simulink model "main"  (R2018a)
settings: Solver=VariableStepAuto  StartTime=0.0  StopTime=10  RelTol=1e-3
libraries: simulink x2
settings Model: Creator=user  LastModifiedBy=user

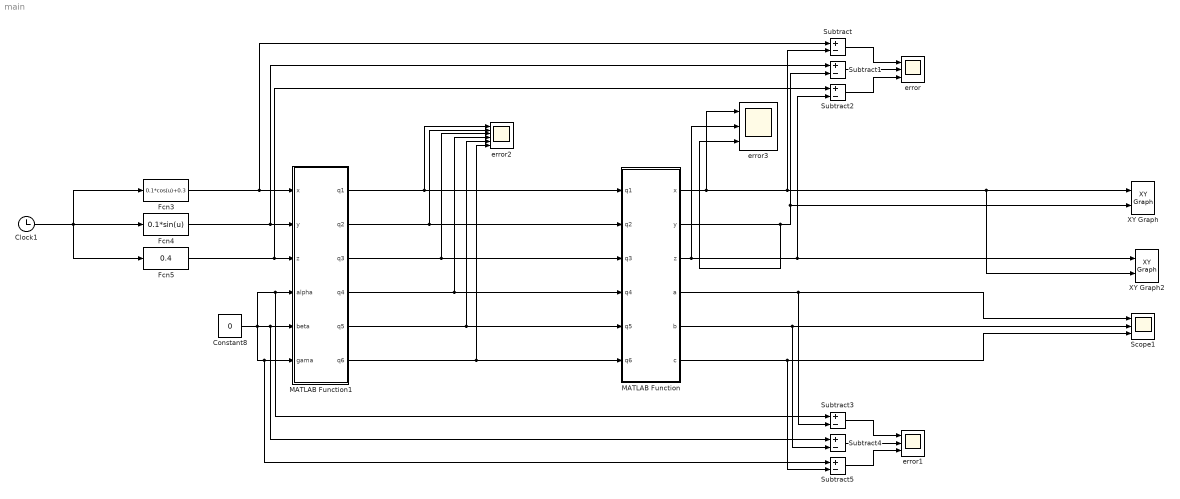
== system main ==
  Clock1 : Clock
  Constant8 : Constant  Value=0
  Fcn3 : Fcn  Expr=0.1*cos(u)+0.3
  Fcn4 : Fcn  Expr=0.1*sin(u)
  Fcn5 : Fcn  Expr=0.4
  MATLAB Function : MATLAB Function  TreatAsAtomicUnit=on
  MATLAB Function1 : MATLAB Function  TreatAsAtomicUnit=on
  Scope1 : Scope  NumInputPorts=3
  Subtract{,1..5} (6 alike) : Sum  Inputs=+-
  XY Graph : simulink/Sinks/XY Graph  xmin=-2  xmax=2  ymin=-2  ymax=2  st=-1
  XY Graph2 : simulink/Sinks/XY Graph  xmin=-2  xmax=2  ymin=-2  ymax=2  st=-1
  error : Scope  NumInputPorts=3
  error1 : Scope  NumInputPorts=3
  error2 : Scope  NumInputPorts=6
  error3 : Scope  NumInputPorts=3
  wires:
  Constant8/1 -> MATLAB Function1/4(alpha), Subtract3/1, MATLAB Function1/6(gama), Subtract5/1, MATLAB Function1/5(beta), Subtract4/1
  MATLAB Function/1(x) -> error3/1, Subtract/2, XY Graph2/2, XY Graph/1
  MATLAB Function/2(y) -> error3/3, Subtract1/2, XY Graph/2
  MATLAB Function/3(z) -> error3/2, XY Graph2/1, Subtract2/2
  MATLAB Function/4(a) -> Subtract3/2, Scope1/1
  MATLAB Function/5(b) -> Subtract4/2, Scope1/2
  MATLAB Function/6(c) -> Subtract5/2, Scope1/3
  MATLAB Function1/1(q1) -> error2/1, MATLAB Function/1(q1)
  Subtract/1 -> error/1
  Subtract1/1 -> error/2
  Subtract2/1 -> error/3
  Subtract5/1 -> error1/3
  Subtract4/1 -> error1/2
  Subtract3/1 -> error1/1
  MATLAB Function1/2(q2) -> error2/2, MATLAB Function/2(q2)
  MATLAB Function1/3(q3) -> error2/3, MATLAB Function/3(q3)
  MATLAB Function1/4(q4) -> error2/4, MATLAB Function/4(q4)
  MATLAB Function1/5(q5) -> error2/5, MATLAB Function/5(q5)
  Clock1/1 -> Fcn3/1, Fcn4/1, Fcn5/1
  MATLAB Function1/6(q6) -> error2/6, MATLAB Function/6(q6)
  Fcn3/1 -> Subtract/1, MATLAB Function1/1(x)
  Fcn4/1 -> Subtract1/1, MATLAB Function1/2(y)
  Fcn5/1 -> Subtract2/1, MATLAB Function1/3(z)

== matlab function main/MATLAB Function ==
  data: q1 input; x output; y output; z output; a output; b output; c output; q2 input; q3 input; q4 input; q5 input; q6 input
function [x,y,z,a,b,c] = FK(q1,q2,q3,q4,q5,q6)

% -------------DH_Parametrs--------------------
a0 = 0;     d1 = 0.352;      alpha0 = 0;
a1 = 0.07;    d2 = 0;        alpha1 = -pi/2;
a2 = 0.36;   d3 = 0;        alpha2 = 0;
a3 = 0;     d4 = 0.380;      alpha3 = -pi/2;
a4 = 0;     d5 = 0;        alpha4 = pi/2;
a5 = 0;     d6 = 0;        alpha5 = -pi/2;

theta1 =q1;
theta2 =q2;
theta3 =q3;
theta4 =q4; 
theta5 =q5;
theta6 =q6;


T10 = DHFUNCTION(a0,alpha0,d1,theta1);
T21 = DHFUNCTION(a1,alpha1,d2,(theta2-pi/2));
T32 = DHFUNCTION(a2,alpha2,d3,theta3);
T43 = DHFUNCTION(a3,alpha3,d4,theta4);
T54 = DHFUNCTION(a4,alpha4,d5,theta5);
T65 = DHFUNCTION(a5,alpha5,d6,theta6);

T20 = T10*T21;
T30 = T20*T32;
T64 = T54*T65;
T63 = T43*T64;
T60 = T30*T63;


Xw = T60(1,4);
Yw = T60(2,4);
Zw = T60(3,4);

P6 = [Xw;Yw;Zw];

PTCP= T60*[0;0;0.065;1];

x=PTCP(1);
y=PTCP(2);
z=PTCP(3);

a=atan2(sqrt(1-(T60(1,3)/sqrt(T60(1,3)^2+T60(2,3)^2+T60(3,3)^2))^2),T60(1,3)/sqrt(T60(1,3)^2+T60(2,3)^2+T60(3,3)^2));
b=atan2(sqrt(1-(T60(1,3)/sqrt(T60(1,3)^2+T60(2,3)^2+T60(3,3)^2))^2),T60(2,3)/sqrt(T60(1,3)^2+T60(2,3)^2+T60(3,3)^2));
c=atan2(sqrt(1-(T60(1,3)/sqrt(T60(1,3)^2+T60(2,3)^2+T60(3,3)^2))^2),T60(3,3)/sqrt(T60(1,3)^2+T60(2,3)^2+T60(3,3)^2));

function T = DHFUNCTION(ai,alphai,di,thetai)

T = [ cos(thetai), -1.*sin(thetai), 0, ai ;
 sin(thetai).*cos(alphai), cos(thetai).*cos(alphai), -1.*sin(alphai), 1*di.*sin(alphai);
 sin(thetai).*sin(alphai), cos(thetai).*sin(alphai), cos(alphai), di.*cos(alphai);
 0, 0, 0, 1 ];

end
end

== matlab function main/MATLAB Function1 ==
  data: x input; q1 output; y input; z input; alpha input; beta input; gama input; q2 output; q3 output; q4 output; q5 output; q6 output
function [q1,q2,q3,q4,q5,q6] = IK_IRB140(x,y,z,alpha,beta,gama) 
% x=0.3;
% y=0.3;
% z=0.2;
% alpha=0;
% beta=0;
% gama=0;

d1 = 0.352;
a1 = 0.070;
a2 = 0.360;
d4 = 0.380;
d6=0.065;
q1=0;
q2=0;
q3=0;
q4=0;
q5=0;
q6=0;

NOSOLUTION=1000;

Q1= atan2 (y,x);
Q11= pi + Q1;


s = (z - d1);
r = sqrt((x - a1*cos (Q1))^2 +(y - a1*sin(Q1))^2);
czeta = (r^2 + s^2 - (a2)^2 - (d4 + d6)^2)/(2 * a2 *(d4 + d6));
    szeta = sqrt(1-(czeta)^2);
    szeta1 = -szeta;
    zeta= atan2(szeta,czeta);
    zeta1= atan2(szeta1,czeta);
if (abs(czeta) <= 1)
  
    Q3 = -(pi/2 + zeta);
    Q33 = -(pi/2 + zeta1);
    Q3 = conversion( Q3,50,-230);
    Q33 = conversion( Q33,50,-230);
else
    Q3 = NOSOLUTION; 
    Q33= NOSOLUTION;
end


s = (z - d1);
r = sqrt((x - a1*cos (Q11))^2 +(y - a1*sin(Q11))^2);
czetai = (r^2 + s^2 - (a2)^2 - (d4 + d6)^2)/(2 * a2 *(d4 + d6));
    
    szetai = sqrt(1-(czetai)^2);
    szeta1i = -szetai;
    zetai= atan2(szetai,czetai);
    zeta1i= atan2(szeta1i,czetai);
if (abs(czetai) <= 1)
   
    Q3i = -(pi/2 + zetai);
    Q33i = -(pi/2 + zeta1i);
    Q3i = conversion( Q3i,50,-230);
    Q33i = conversion( Q33i,50,-230);
else
    Q3i=NOSOLUTION;
    Q33i=NOSOLUTION; 
end




if (Q3 == NOSOLUTION)
    Q2 = NOSOLUTION;
    Q22 = NOSOLUTION;
else
    Q2 = THE2(x,y,z,Q1,zeta);
    Q22 = THE2COMP(x,y,z,Q1,zeta);
    Q2 = conversion( Q2,110,-90);
    Q22 = conversion( Q22,110,-90);
end



if (Q33 == NOSOLUTION)
    Q2i = NOSOLUTION;
    Q22i = NOSOLUTION;
else
    Q2i = THE2(x,y,z,Q1,zeta1);
    Q22i = THE2COMP(x,y,z,Q1,zeta1);
    Q2i = conversion( Q2i,110,-90);
    Q22i = conversion( Q22i,110,-90);
end

if (Q3i == NOSOLUTION)
    Q2j = NOSOLUTION;
    Q22j = NOSOLUTION;
else
    Q2j = THE2(x,y,z,Q11,zetai); 
    Q22j = THE2COMP(x,y,z,Q11,zetai);
    Q2j = conversion( Q2j,100,-90);
    Q22j = conversion( Q22j,100,-90);
end



if (Q33i == NOSOLUTION)
    Q2k = NOSOLUTION;
    Q22k = NOSOLUTION;
else
    Q2k = THE2(x,y,z,Q11,zeta1i);
    Q22k = THE2COMP(x,y,z,Q11,zeta1i);
    Q2k = conversion( Q2k,110,-90);
    Q22k = conversion( Q22k,110,-90);
end


SOL1 =[ Q1, Q2, Q3];
SOL2 =[ Q1, Q22,Q3];
SOL3 =[ Q1, Q2i, Q33];
SOL4 =[ Q1, Q22i, Q33];
SOL5 =[ Q11, Q2j, Q3i];
SOL6 =[ Q11, Q22j, Q3i];
SOL7 =[ Q11, Q2k, Q33i];
SOL8 =[ Q11, Q22k, Q33i];

SOLUTION=[SOL1;SOL2;SOL3;SOL4;SOL5;SOL6;SOL7;SOL8];

for i=1:length(SOLUTION)
    if max(SOLUTION(i,1:end))~=NOSOLUTION
    q1=SOLUTION(i,1);
    q2=SOLUTION(i,2);
    q3=SOLUTION(i,3);
    break
    end
end

R60 = [cos(alpha).*cos(beta), (cos(alpha).*sin(beta).*sin(gama))- sin(alpha).*cos(gama),(cos(alpha).*sin(beta).*cos(gama)) + sin(alpha).*sin(gama) ;
 sin(alpha).*cos(beta), (sin(alpha).*sin(beta).*sin(gama)) + cos(alpha).*cos(gama),(sin(alpha).*sin(beta).*cos(gama)) - cos(alpha).*sin(gama) ;
 - sin(beta), cos(beta).*sin(gama), cos(beta).*sin(gama)];
R30 = [cos(q1).*cos(q2+q3), -cos(q1).*sin(q2+q3), sin(q1);
 sin(q1).*cos(q2+q3), -sin(q1).*sin(q2+q3), cos(q1);
 -sin(q2+q3), -cos(q2+q3), 0 ] ;
 
RT30= transpose (R30);
R63 = RT30 * R60 ;
g11 = R63 (1,1);
g12 = R63 (1,2);
g23 = R63 (2,3);
g31 = R63 (3,1);
g32 = R63 (3,2);
g33 = R63 (3,3);


Q5 = atan2 ( sqrt((g31)^2 +(g32)^2), g33);
if(Q5 == 0)
    q4= 0;
    q5= 0;
    q6 = atan2 (-g12, g11);
elseif (Q5 == pi)
    q4= 0;
    q5= 0;
    q6 = atan2 (g12,-g11);
else
    Q4 = atan2 (g32/ sin (Q5), - g31/ sin (Q5));
    Q6 = atan2 (g23/ sin (Q5), g31/ sin (Q5));
    Q4= conversion( Q4,200,-200);
    Q5= conversion( Q5,115,-115);
    Q6= conversion( Q6,400,-400);


    Q44 = Q4 + pi;
    Q55 = -Q5;
    Q66 = Q6+pi;
    Q44= conversion( Q44,200,-200);
    Q55= conversion( Q55,115,-115);
    Q66= conversion( Q66,400,-400);

    Solution1 = [Q4,Q5,Q6];
    Solution2 = [Q44,Q55,Q66];
    
    SOLUTION2=[Solution1;Solution2];
    for i=1:2
        if max(SOLUTION2(i,1:end))~=NOSOLUTION
            q4=SOLUTION2(i,1);
            q5=SOLUTION2(i,2);
            q6=SOLUTION2(i,3);
            break
        end
    end
end





function RES = THE2(xtip,ytip,ztip,theta1,zeta)
    s = (ztip - d1);
    r = sqrt((xtip - a1*cos (theta1))^2 +(ytip - a1*sin(theta1))^2);
    omega = atan2 (s, r);
    lenda = atan2 (( d4+d6) * sin (zeta) , a2+( d4+d6)* cos (zeta));
    RES = - ((omega - lenda)- ( pi/2)) ;
end


function RES1 = THE2COMP(xtip,ytip,ztip,theta1,zeta)
    s = (ztip - d1);
    r = - sqrt((xtip - a1*cos (theta1))^2 +(ytip - a1*sin(theta1))^2);
    omega = atan2 (s, r);
    lenda = atan2 (( d4+d6) * sin (zeta) , a2+( d4+d6)* cos (zeta));
    RES1 = - ((omega - lenda) - ( pi/2));
end

function OUT = conversion( theta,upperlimit,lowerlimit)
    upperlimit = upperlimit * pi / 180;
    lowerlimit = lowerlimit * pi / 180;
    if (theta > upperlimit)
        OUT = NOSOLUTION;
    elseif (theta < lowerlimit)
        OUT = NOSOLUTION;
    else
        OUT = theta;
    end
end
end
